simulink model "eventdemux_plots"  (R2022a)
settings: Solver=VariableStepAuto  StartTime=0.0  StopTime=10.0  RelTol=1e-3
libraries: neuromorphic_blocks x5
settings Model: Creator=chris  LastModifiedBy=chris

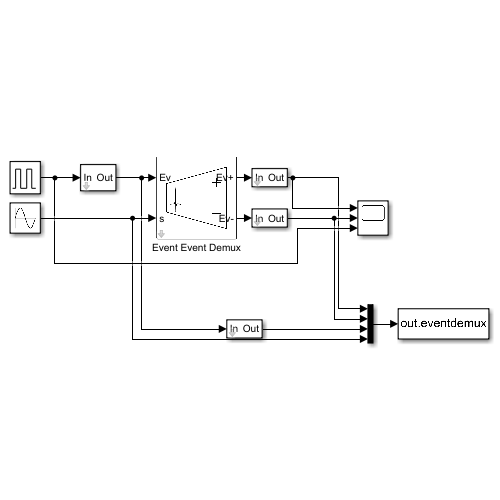
[thumbnail: Simulink's stored preview of the top-level diagram]
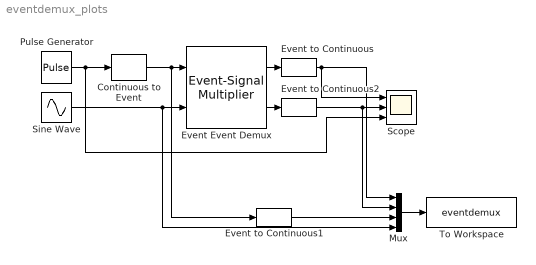
== system eventdemux_plots ==
  Continuous to Event : neuromorphic_blocks/Events Transmission Blocks/Continuous to Event  thresh=5
      settings: SourceProductName=Neuromorphic Toolbox
  Event Event Demux : neuromorphic_blocks/Auxiliary Blocks/Event-Signal Multiplier  symmetric_box=off  dsyn_signal_pos=0  dsyn_signal_neg=0  dsyn_signal_neg_save=0  gain_signal_pos=10  gain_signal_neg=10  gain_signal_neg_save=10  input=Events  gsyn_pos=10  gsyn_neg=10  gsyn_neg_save=10  dsyn_event_pos=5  dsyn_event_neg=5  dsyn_event_neg_save=5  gain_event_pos=20  gain_event_neg=20  gain_event_neg_save=20
      settings: SourceProductName=NeurCont Toolbox
  Event to Continuous : neuromorphic_blocks/Events Transmission Blocks/Event to Continuous  gain=1
      settings: SourceProductName=Neuromorphic Toolbox
  Event to Continuous1 : neuromorphic_blocks/Events Transmission Blocks/Event to Continuous  gain=1
      settings: SourceProductName=Neuromorphic Toolbox
  Event to Continuous2 : neuromorphic_blocks/Events Transmission Blocks/Event to Continuous  gain=1
      settings: SourceProductName=Neuromorphic Toolbox
  Mux : Mux
  Pulse Generator : DiscretePulseGenerator  PulseType=Time based  Amplitude=20  Period=0.3  PulseWidth=5
  Scope : Scope  NumInputPorts=3
  Sine Wave : Sin  SampleTime=0
  To Workspace : ToWorkspace  VariableName=eventdemux  SaveFormat=Structure With Time  SampleTime=0.001
  wires:
  Pulse Generator/1 -> Continuous to Event/1, Scope/3
  Sine Wave/1 -> Event Event Demux/2, Mux/4
  Event Event Demux/1 -> Event to Continuous/1
  Event Event Demux/2 -> Event to Continuous2/1
  Mux/1 -> To Workspace/1
  Continuous to Event/1 -> Event Event Demux/1, Event to Continuous1/1
  Event to Continuous1/1 -> Mux/3
  Event to Continuous/1 -> Scope/1, Mux/1
  Event to Continuous2/1 -> Scope/2, Mux/2
